simulink model "simulinkFLC_v1"  (R2016a)
settings: Solver=VariableStepAuto  StartTime=0.0  StopTime=10.0  RelTol=1e-3
undefined symbols (not defined in the file): FLC_v2
libraries: fuzblock x1
settings Model: Creator=PC  LastModifiedBy=PC

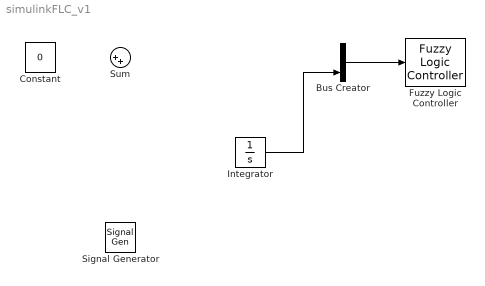
== system simulinkFLC_v1 ==
  Bus Creator : BusCreator  Inputs=2
  Constant : Constant  Value=0
  Fuzzy Logic Controller : fuzblock/Fuzzy Logic  Controller  fis=[FLC_v2.fis]
  Integrator : Integrator
  Signal Generator : SignalGenerator  Units=rad/sec
  Sum : Sum  Inputs=|++
  wires:
  Bus Creator/1 -> Fuzzy Logic Controller/1
  Integrator/1 -> Bus Creator/2
